simulink subsystem "altitude_control"  (R2020a)
settings: Solver=VariableStepAuto  StartTime=0.0  StopTime=10.0  RelTol=1e-3
values from neighbouring files (symbols this model uses):
  Kd = 1e-1    (= 0.1)    [ascent_model_variable_mass.m]
  Ki = 1.5e-10    [ascent_model_variable_mass.m]
  Kn = 1e-0    (= 1)    [ascent_model_variable_mass.m]
  Kp = 5e-1    (= 0.5)    [ascent_model_variable_mass.m]
  mdot_ballast_max = 0.010    (= 0.01)    [ascent_model_variable_mass.m]
  mdot_ballast_min = 0.001    [ascent_model_variable_mass.m]
  mdot_bleed_max = 0.010    (= 0.01)    [ascent_model_variable_mass.m]
libraries: simulink x6
settings Model: Creator=Philip  LastModifiedBy=Philip

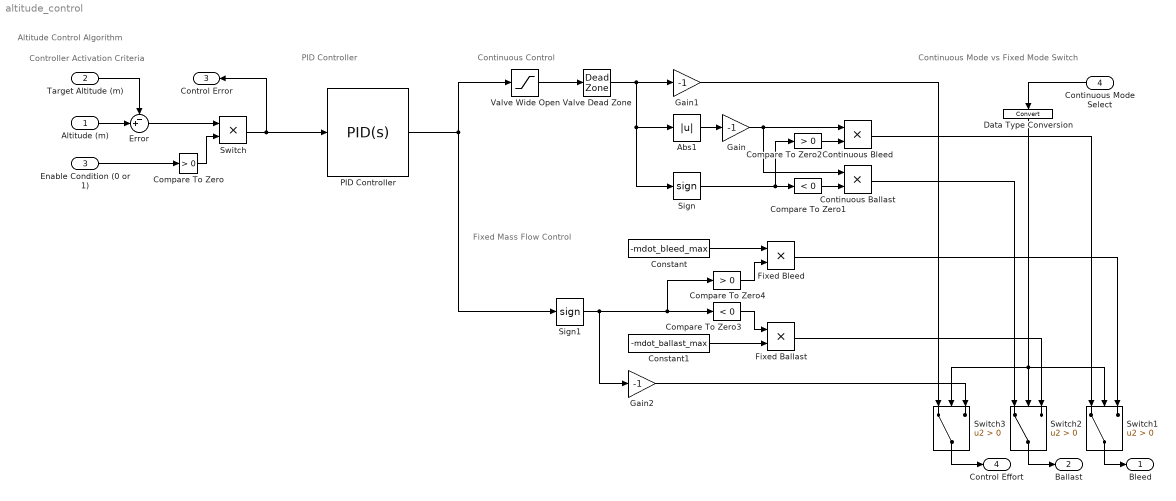
== system altitude_control ==
  note: Continuous Mode vs Fixed Mode Switch
  note: Fixed Mass Flow Control
  note: Altitude Control Algorithm
  note: Controller Activation Criteria
  note: PID Controller
  note: Continuous Control
  Altitude (m) : Inport
  Target Altitude (m) : Inport  Port=2
  Enable Condition (0 or 1) : Inport  Port=3
  Continuous Mode Select : Inport  Port=4
  Abs1 : Abs
  Compare To Zero : simulink/Logic and Bit Operations/Compare To Zero  relop=>  OutDataTypeStr=uint8
  Compare To Zero1 : simulink/Logic and Bit Operations/Compare To Zero  relop=<  OutDataTypeStr=uint8
  Compare To Zero2 : simulink/Logic and Bit Operations/Compare To Zero  relop=>  OutDataTypeStr=uint8
  Compare To Zero3 : simulink/Logic and Bit Operations/Compare To Zero  relop=<  OutDataTypeStr=uint8
  Compare To Zero4 : simulink/Logic and Bit Operations/Compare To Zero  relop=>  OutDataTypeStr=uint8
  Constant : Constant  Value=-mdot_bleed_max
  Constant1 : Constant  Value=-mdot_ballast_max
  Continuous Ballast : Product
  Continuous Bleed : Product
  Data Type Conversion : DataTypeConversion
  Error : Sum  Inputs=-+|
  Fixed Ballast : Product
  Fixed Bleed : Product
  Gain : Gain  Gain=-1
  Gain1 : Gain  Gain=-1
  Gain2 : Gain  Gain=-1
  PID Controller : simulink/Continuous/PID Controller  Controller=PID  Form=Parallel  TimeDomain=Continuous-time  UseExternalTs=off  SampleTime=-1  IntegratorMethod=Forward Euler  FilterMethod=Forward Euler  ControllerParametersSource=internal  P=Kp  I=Ki  D=Kd  UseFilter=on  N=Kn  TunerSelectOption=Transfer Function Based (PID Tuner App)  InitialConditionSource=internal  InitialConditionForIntegrator=0  InitialConditionForFilter=0  DifferentiatorICPrevScaledInput=0  ExternalReset=none  TrackingMode=off  Kt=1  LimitOutput=on  UpperSaturationLimit=mdot_bleed_max  LowerSaturationLimit=-mdot_ballast_max  LinearizeAsGain=on  AntiWindupMode=none  Kb=1  POutMin=[]  POutMax=[]  IOutMin=[]  IOutMax=[]  DOutMin=[]  DOutMax=[]  NOutMin=[]  NOutMax=[]  SumOutMin=[]  SumOutMax=[]  SaturationOutMin=[]  SaturationOutMax=[]  PParamMin=[]  PParamMax=[]  IParamMin=[]  IParamMax=[]  DParamMin=[]  DParamMax=[]  NParamMin=[]  NParamMax=[]  KbParamMin=[]  KbParamMax=[]  KtParamMin=[]  KtParamMax=[]  KbOutMin=[]  KbOutMax=[]  KtOutMin=[]  KtOutMax=[]  IntegratorOutMin=[]  IntegratorOutMax=[]  FilterOutMin=[]  FilterOutMax=[]  SumI1OutMin=[]  SumI1OutMax=[]  SumI2OutMin=[]  SumI2OutMax=[]  SumI3OutMin=[]  SumI3OutMax=[]  SumI4OutMin=[]  SumI4OutMax=[]  SumDOutMin=[]  SumDOutMax=[]  DifferentiatorOutMin=[]  DifferentiatorOutMax=[]  FilterDiffOutCoefMin=[]  FilterDiffOutCoefMax=[]  ReciprocalOutMin=[]  ReciprocalOutMax=[]  SumDenOutMin=[]  SumDenOutMax=[]  SumNumOutMin=[]  SumNumOutMax=[]  DivideOutMin=[]  DivideOutMax=[]  UdiffTsProdOutMin=[]  UdiffTsProdOutMax=[]  NTsProdOutMin=[]  NTsProdOutMax=[]  UintegralTsProdOutMin=[]  UintegralTsProdOutMax=[]  UngainTsProdOutMin=[]  UngainTsProdOutMax=[]  IntegratorContinuousStateAttributes=''  IntegratorStateMustResolveToSignalObject=off  IntegratorRTWStateStorageClass=Auto  FilterContinuousStateAttributes=''  FilterStateMustResolveToSignalObject=off  FilterRTWStateStorageClass=Auto  ParallelPVariant=InternalParameters  IdealPVariant=Disabled  IVariant=InternalParameters  DVariant=InternalParameters  IntegratorVariant=Continuous  SatVariant=Disabled  AWVariant=Passthrough  PCopyVariant=Disabled  TRVariant=Disabled  FdbkBlocksVariant=Forward  IdealPFdbkVariant=Disabled  SatFdbkVariant=Disabled  DerivativeFilterVariant=ContFilter  NVariant=InternalParameters  NCopyVariant=Disabled  FilterICVariant=InternalICsFilter  IntegratorICVariant=InternalICs  ExternalResetVariant=Disabled  TRSumVariant=Passthrough  SumFdbkVariant=Disabled  SumVariant=Sum_PID  TsampFilterVariant=InternalTs  TsampNgainVariant=Passthrough  TsampIntegralVariant=Passthrough
  Sign : Signum
  Sign1 : Signum
  Switch : Product
  Switch1 : Switch  Criteria=u2 > Threshold
  Switch2 : Switch  Criteria=u2 > Threshold
  Switch3 : Switch  Criteria=u2 > Threshold
  Valve Dead Zone : DeadZone  LowerValue=-mdot_ballast_min  UpperValue=mdot_bleed_min  SaturateOnIntegerOverflow=on
  Valve Wide Open : Saturate  UpperLimit=mdot_bleed_max  LowerLimit=-mdot_ballast_max
  Bleed : Outport
  Ballast : Outport  Port=2
  Control Error : Outport  Port=3
  Control Effort : Outport  Port=4
  wires:
  Compare To Zero1/1 -> Continuous Ballast/2
  Compare To Zero2/1 -> Continuous Bleed/2
  Abs1/1 -> Gain/1
  Compare To Zero/1 -> Switch/2
  Target Altitude (m)/1 -> Error/1
  Altitude (m)/1 -> Error/2
  Error/1 -> Switch/1
  Switch/1 -> PID Controller/1, Control Error/1
  Valve Wide Open/1 -> Valve Dead Zone/1
  Gain/1 -> Continuous Ballast/1, Continuous Bleed/1
  Sign/1 -> Compare To Zero1/1, Compare To Zero2/1
  Valve Dead Zone/1 -> Gain1/1, Abs1/1, Sign/1
  Enable Condition (0 or 1)/1 -> Compare To Zero/1
  PID Controller/1 -> Valve Wide Open/1, Sign1/1
  Compare To Zero3/1 -> Fixed Ballast/1
  Compare To Zero4/1 -> Fixed Bleed/2
  Fixed Bleed/1 -> Switch1/3
  Fixed Ballast/1 -> Switch2/3
  Sign1/1 -> Compare To Zero3/1, Compare To Zero4/1, Gain2/1
  Constant/1 -> Fixed Bleed/1
  Constant1/1 -> Fixed Ballast/2
  Gain1/1 -> Switch3/1
  Gain2/1 -> Switch3/3
  Switch3/1 -> Control Effort/1
  Switch2/1 -> Ballast/1
  Switch1/1 -> Bleed/1
  Continuous Bleed/1 -> Switch1/1
  Continuous Ballast/1 -> Switch2/1
  Continuous Mode Select/1 -> Data Type Conversion/1
  Data Type Conversion/1 -> Switch2/2, Switch3/2, Switch1/2
